simulink model "UPNRZ_UPRZ_BPNRZ_BPRZ"  (R2018a)
settings: Solver=VariableStepAuto  StartTime=0.0  StopTime=50  RelTol=1e-3
libraries: commutil2 x1, commrandsrc3 x1
settings Model: Creator=Souhardhya Paul  LastModifiedBy=Souhardhya Paul

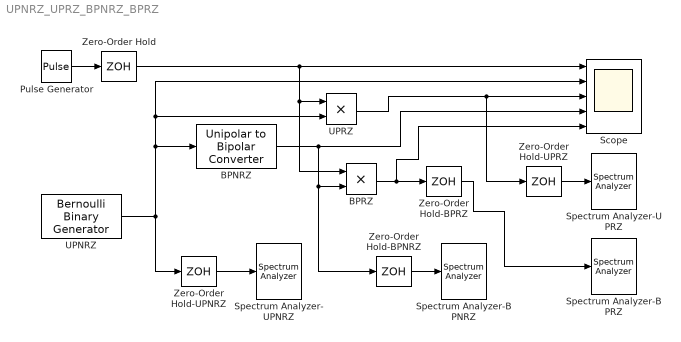
== system UPNRZ_UPRZ_BPNRZ_BPRZ ==
  BPNRZ : commutil2/Unipolar to Bipolar Converter  M=2  polarity=Positive  dataType=Inherit via internal rule
      settings: SourceProductName=Communications System Toolbox
  BPRZ : Product
  Pulse Generator : DiscretePulseGenerator  PulseType=Time based  Period=0.1  PulseWidth=50  SampleTime=0.1
  Scope : Scope  NumInputPorts=5
  Spectrum Analyzer- UPNRZ : SpectrumAnalyzer
  Spectrum Analyzer-BPNRZ : SpectrumAnalyzer
  Spectrum Analyzer-BPRZ : SpectrumAnalyzer
  Spectrum Analyzer-UPRZ : SpectrumAnalyzer
  UPNRZ : commrandsrc3/Bernoulli Binary Generator  ProbabilityOfZero=0.5  SeedSource=Auto  Seed=0  SampleTime=0.1  SamplesPerFrame=1  OutputDataType=boolean  SimulateUsing=Interpreted execution
  UPRZ : Product
  Zero-Order Hold : ZeroOrderHold  SampleTime=0.05
  Zero-Order Hold-BPNRZ : ZeroOrderHold  SampleTime=0.01
  Zero-Order Hold-BPRZ : ZeroOrderHold  SampleTime=0.01
  Zero-Order Hold-UPNRZ : ZeroOrderHold  SampleTime=0.01
  Zero-Order Hold-UPRZ : ZeroOrderHold  SampleTime=0.01
  wires:
  UPNRZ/1 -> BPNRZ/1, Scope/2, UPRZ/2, Zero-Order Hold-UPNRZ/1
  Pulse Generator/1 -> Zero-Order Hold/1
  Zero-Order Hold/1 -> Scope/1, UPRZ/1, BPRZ/1
  BPRZ/1 -> Scope/5, Zero-Order Hold-BPRZ/1
  BPNRZ/1 -> Scope/4, Zero-Order Hold-BPNRZ/1, BPRZ/2
  Zero-Order Hold-BPNRZ/1 -> Spectrum Analyzer-BPNRZ/1
  UPRZ/1 -> Zero-Order Hold-UPRZ/1, Scope/3
  Zero-Order Hold-BPRZ/1 -> Spectrum Analyzer-BPRZ/1
  Zero-Order Hold-UPNRZ/1 -> Spectrum Analyzer- UPNRZ/1
  Zero-Order Hold-UPRZ/1 -> Spectrum Analyzer-UPRZ/1
